simulink model "ModelR3"  (R2020a)
settings: Solver=FixedStepAuto  StartTime=0.0  StopTime=Tf  FixedStep=0.1  RelTol=1e-3
undefined symbols (not defined in the file): amax_ego, amin_ego, d_target, t_gap, Tf, Ts, v0_ego, v0_lead, x0_ego, x0_lead
libraries: simulink x6, rllib x1
settings Model: Creator=The MathWorks, Inc.  LastModifiedBy=kn944
settings DataIOCC: ReturnWorkspaceOutputs=off
settings DebuggingCC: ArithmeticOperatorsInVariantConditions=warning
settings SFSimCC: SimUseLocalCustomCode=off
settings RTWCC: RTWUseLocalCustomCode=off
settings CodeAppCC: StateflowObjectComments=on

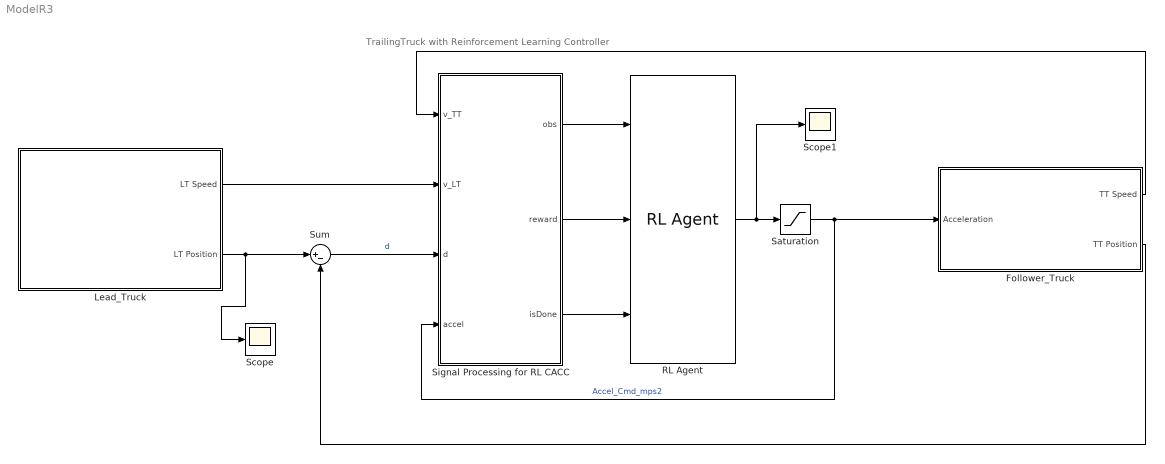
== system ModelR3 ==
  note: TrailingTruck with Reinforcement Learning Controller
  Follower_Truck : Subsystem
  Lead_Truck : Subsystem
  RL Agent : rllib/RL Agent  Agent=agent  ProvideReward=on  ProvideIsDone=on  ProvideCumRwd=off  TreatAsDirectFeedthrough=on  CollectLoggedSignals=on  CollectModelStates=on
  Saturation : Saturate  UpperLimit=amax_ego  LowerLimit=amin_ego
  Scope : Scope
  Scope1 : Scope
  Signal Processing for RL CACC : Subsystem
  Sum : Sum  Inputs=|+-
  wires:
  Signal Processing for RL CACC/2(reward) -> RL Agent/2
  Signal Processing for RL CACC/3(isDone) -> RL Agent/3
  Signal Processing for RL CACC/1(obs) -> RL Agent/1
  Sum/1 -> Signal Processing for RL CACC/3(d)  "d"
  Saturation/1 -> Signal Processing for RL CACC/4(accel), Follower_Truck/1(Acceleration)  "Accel_Cmd_mps2"
  Lead_Truck/1(LT Speed) -> Signal Processing for RL CACC/2(v_LT)
  Lead_Truck/2(LT Position) -> Scope/1, Sum/1
  Follower_Truck/1(TT Speed) -> Signal Processing for RL CACC/1(v_TT)
  Follower_Truck/2(TT Position) -> Sum/2
  RL Agent/1 -> Scope1/1, Saturation/1

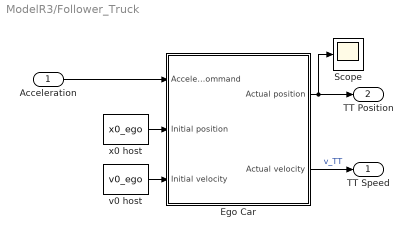
== system ModelR3/Follower_Truck ==
  Acceleration : Inport
  Ego Car : Subsystem
  Scope : Scope
  v0 host : Constant  Value=v0_ego  SampleTime=Ts
  x0 host : Constant  Value=x0_ego  SampleTime=Ts
  TT Speed : Outport
  TT Position : Outport  Port=2
  wires:
  Ego Car/1(Actual position) -> TT Position/1, Scope/1
  x0 host/1 -> Ego Car/2(Initial position)
  v0 host/1 -> Ego Car/3(Initial velocity)
  Ego Car/2(Actual velocity) -> TT Speed/1  "v_TT"
  Acceleration/1 -> Ego Car/1(Acceleration Command)

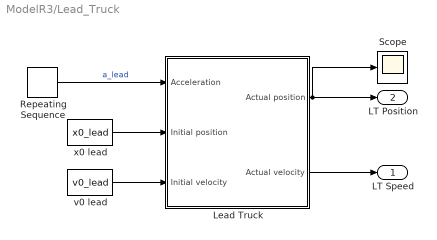
== system ModelR3/Lead_Truck ==
  Lead Truck : Subsystem
  Repeating Sequence : simulink/Sources/Repeating Sequence  rep_seq_t=[0 5 5.1 8 8.1 15 15.1 17 17.1 25]  rep_seq_y=[0 0 0.8 0.8 0 0 -2 -2 0 0]
  Scope : Scope
  v0 lead : Constant  Value=v0_lead  SampleTime=Ts
  x0 lead : Constant  Value=x0_lead  SampleTime=Ts
  LT Speed : Outport
  LT Position : Outport  Port=2
  wires:
  Repeating Sequence/1 -> Lead Truck/1(Acceleration)  "a_lead"
  x0 lead/1 -> Lead Truck/2(Initial position)
  v0 lead/1 -> Lead Truck/3(Initial velocity)
  Lead Truck/2(Actual velocity) -> LT Speed/1
  Lead Truck/1(Actual position) -> Scope/1, LT Position/1

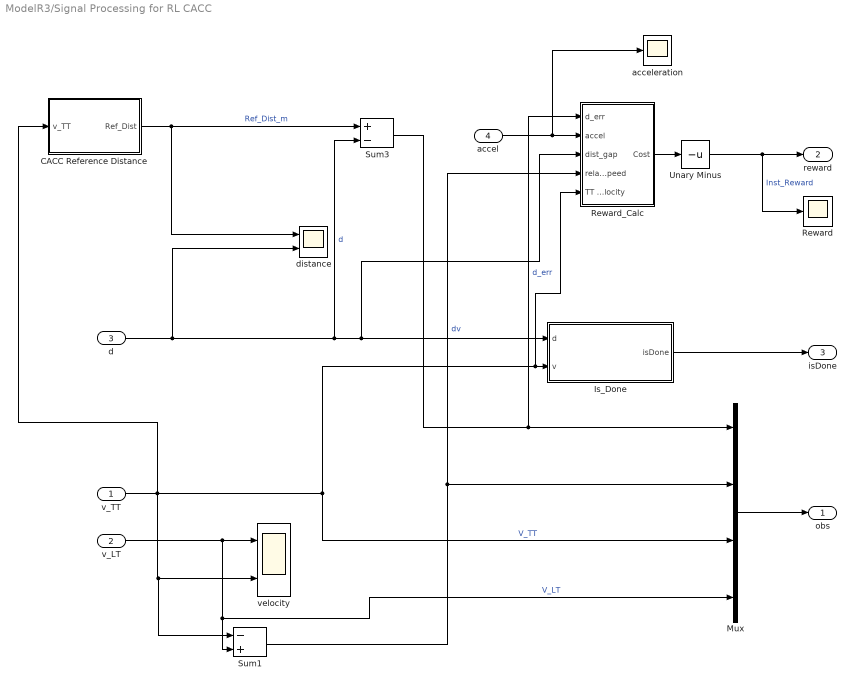
== system ModelR3/Signal Processing for RL CACC ==
  v_TT : Inport
  v_LT : Inport  Port=2
  d : Inport  Port=3
  accel : Inport  Port=4
  CACC Reference Distance : Subsystem
  Is_Done : Subsystem
  Mux : Mux
  Reward : Scope
  Reward_Calc : Subsystem
  Sum1 : Sum  Inputs=-+
  Sum3 : Sum  Inputs=+-
  Unary Minus : UnaryMinus
  acceleration : Scope
  distance : Scope  NumInputPorts=2
  velocity : Scope  NumInputPorts=2
  obs : Outport  VectorParamsAs1DForOutWhenUnconnected=off
  reward : Outport  Port=2  VectorParamsAs1DForOutWhenUnconnected=off
  isDone : Outport  Port=3  VectorParamsAs1DForOutWhenUnconnected=off
  wires:
  Mux/1 -> obs/1
  v_TT/1 -> Sum1/1, velocity/2, Mux/3, Reward_Calc/5(TT velocity), Is_Done/2(v), CACC Reference Distance/1(v_TT)  "V_TT"
  d/1 -> Sum3/2, Reward_Calc/3(dist_gap), Is_Done/1(d), distance/2  "d"
  Reward_Calc/1(Cost) -> Unary Minus/1
  Unary Minus/1 -> Reward/1, reward/1  "Inst_Reward"
  Sum3/1 -> Reward_Calc/1(d_err), Mux/1  "d_err"
  accel/1 -> acceleration/1, Reward_Calc/2(accel)
  Is_Done/1(isDone) -> isDone/1
  CACC Reference Distance/1(Ref_Dist) -> Sum3/1, distance/1  "Ref_Dist_m"
  v_LT/1 -> Mux/4, Sum1/2, velocity/1  "V_LT"
  Sum1/1 -> Reward_Calc/4(relative_Speed), Mux/2  "dv"

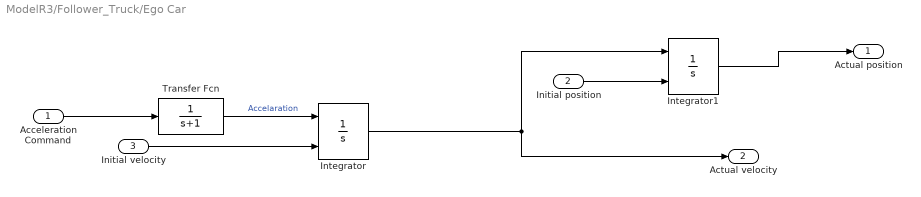
== system ModelR3/Follower_Truck/Ego Car ==
  Acceleration Command : Inport
  Initial position : Inport  Port=2
  Initial velocity : Inport  Port=3
  Integrator : Integrator  InitialConditionSource=external  UpperSaturationLimit=42  LowerSaturationLimit=0
  Integrator1 : Integrator  InitialConditionSource=external  UpperSaturationLimit=500  LowerSaturationLimit=0
  Transfer Fcn : TransferFcn  Denominator=[1 1]
  Actual position : Outport  VectorParamsAs1DForOutWhenUnconnected=off
  Actual velocity : Outport  Port=2  VectorParamsAs1DForOutWhenUnconnected=off
  wires:
  Integrator1/1 -> Actual position/1
  Initial position/1 -> Integrator1/2
  Integrator/1 -> Integrator1/1, Actual velocity/1
  Initial velocity/1 -> Integrator/2
  Transfer Fcn/1 -> Integrator/1  "Accelaration"
  Acceleration Command/1 -> Transfer Fcn/1

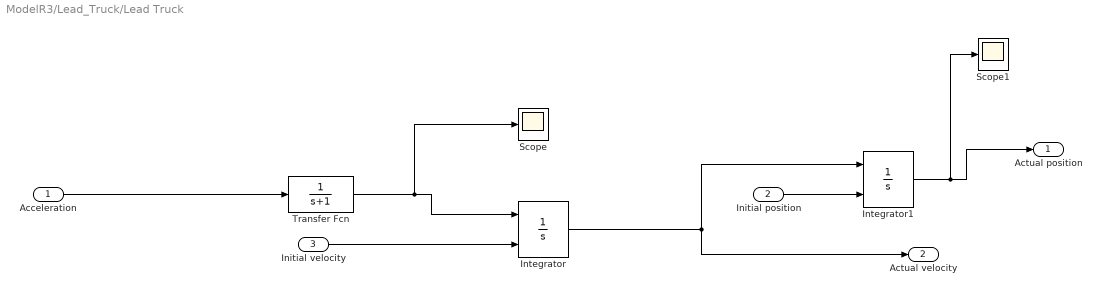
== system ModelR3/Lead_Truck/Lead Truck ==
  Acceleration : Inport
  Initial position : Inport  Port=2
  Initial velocity : Inport  Port=3
  Integrator : Integrator  InitialConditionSource=external  UpperSaturationLimit=40  LowerSaturationLimit=0
  Integrator1 : Integrator  InitialConditionSource=external  UpperSaturationLimit=500  LowerSaturationLimit=0
  Scope : Scope
  Scope1 : Scope
  Transfer Fcn : TransferFcn  Denominator=[1 1]
  Actual position : Outport  VectorParamsAs1DForOutWhenUnconnected=off
  Actual velocity : Outport  Port=2  VectorParamsAs1DForOutWhenUnconnected=off
  wires:
  Integrator1/1 -> Scope1/1, Actual position/1
  Integrator/1 -> Integrator1/1, Actual velocity/1
  Initial velocity/1 -> Integrator/2
  Transfer Fcn/1 -> Scope/1, Integrator/1
  Acceleration/1 -> Transfer Fcn/1
  Initial position/1 -> Integrator1/2

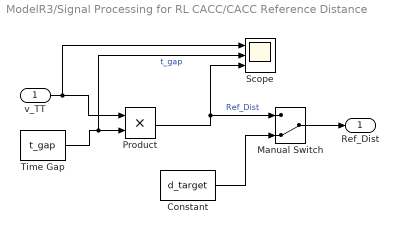
== system ModelR3/Signal Processing for RL CACC/CACC Reference Distance ==
  v_TT : Inport
  Constant : Constant  Value=d_target
  Manual Switch : ManualSwitch  CurrentSetting=0
  Product : Product
  Scope : Scope  NumInputPorts=3
  Time Gap : Constant  Value=t_gap  SampleTime=Ts
  Ref_Dist : Outport  VectorParamsAs1DForOutWhenUnconnected=off
  wires:
  Time Gap/1 -> Scope/2, Product/2  "t_gap"
  Product/1 -> Manual Switch/1, Scope/3  "Ref_Dist"
  v_TT/1 -> Scope/1, Product/1
  Manual Switch/1 -> Ref_Dist/1
  Constant/1 -> Manual Switch/2

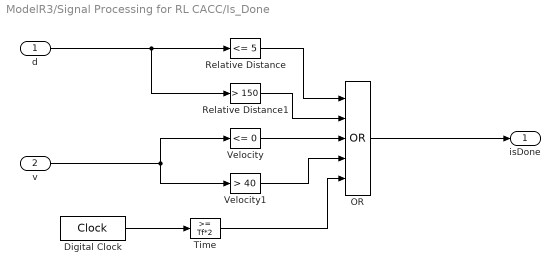
== system ModelR3/Signal Processing for RL CACC/Is_Done ==
  d : Inport
  v : Inport  Port=2
  Digital Clock : DigitalClock
  OR : Logic  Operator=OR  Inputs=5  AllPortsSameDT=off  OutDataTypeStr=boolean
  Relative Distance : simulink/Logic and Bit Operations/Compare To Constant  relop=<=  const=5  OutDataTypeStr=boolean
  Relative Distance1 : simulink/Logic and Bit Operations/Compare To Constant  relop=>  const=150  OutDataTypeStr=boolean
  Time : simulink/Logic and Bit Operations/Compare To Constant  relop=>=  const=Tf*2  OutDataTypeStr=boolean
  Velocity : simulink/Logic and Bit Operations/Compare To Constant  relop=<=  const=0  OutDataTypeStr=boolean
  Velocity1 : simulink/Logic and Bit Operations/Compare To Constant  relop=>  const=40  OutDataTypeStr=boolean
  isDone : Outport  VectorParamsAs1DForOutWhenUnconnected=off
  wires:
  d/1 -> Relative Distance1/1, Relative Distance/1
  v/1 -> Velocity1/1, Velocity/1
  OR/1 -> isDone/1
  Relative Distance/1 -> OR/1
  Relative Distance1/1 -> OR/2
  Velocity/1 -> OR/3
  Velocity1/1 -> OR/4
  Digital Clock/1 -> Time/1
  Time/1 -> OR/5

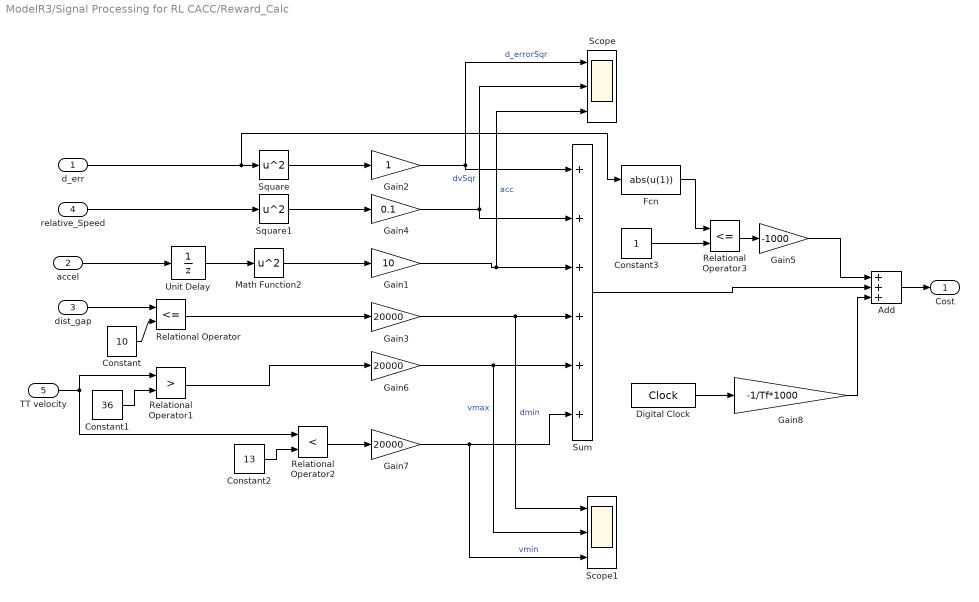
== system ModelR3/Signal Processing for RL CACC/Reward_Calc ==
  d_err : Inport
  accel : Inport  Port=2
  dist_gap : Inport  Port=3
  relative_Speed : Inport  Port=4
  TT velocity : Inport  Port=5
  Add : Sum  Inputs=+++
  Constant : Constant  Value=10
  Constant1 : Constant  Value=36
  Constant2 : Constant  Value=13
  Constant3 : Constant
  Digital Clock : DigitalClock
  Fcn : Fcn  Expr=abs(u(1))
  Gain1 : Gain  Gain=10
  Gain2 : Gain
  Gain3 : Gain  Gain=20000
  Gain4 : Gain  Gain=0.1
  Gain5 : Gain  Gain=-1000
  Gain6 : Gain  Gain=20000
  Gain7 : Gain  Gain=20000
  Gain8 : Gain  Gain=-1/Tf*1000
  Math Function2 : Math  Operator=square  SignedPower=on  SaturateOnIntegerOverflow=on
  Relational Operator : RelationalOperator  Operator=<=  OutDataTypeStr=boolean  RndMeth=Simplest
  Relational Operator1 : RelationalOperator  Operator=>  OutDataTypeStr=boolean  RndMeth=Simplest
  Relational Operator2 : RelationalOperator  Operator=<  OutDataTypeStr=boolean  RndMeth=Simplest
  Relational Operator3 : RelationalOperator  Operator=<=  OutDataTypeStr=boolean  RndMeth=Simplest
  Scope : Scope  NumInputPorts=3
  Scope1 : Scope  NumInputPorts=3
  Square : Math  Operator=square  SignedPower=on  SaturateOnIntegerOverflow=on
  Square1 : Math  Operator=square  SignedPower=on  SaturateOnIntegerOverflow=on
  Sum : Sum  Inputs=++++++
  Unit Delay : UnitDelay  SampleTime=-1  HasFrameUpgradeWarning=on
  Cost : Outport  VectorParamsAs1DForOutWhenUnconnected=off
  wires:
  d_err/1 -> Fcn/1, Square/1
  Math Function2/1 -> Gain1/1
  Square/1 -> Gain2/1
  accel/1 -> Unit Delay/1
  dist_gap/1 -> Relational Operator/1
  Constant/1 -> Relational Operator/2
  Relational Operator/1 -> Gain3/1
  relative_Speed/1 -> Square1/1
  Square1/1 -> Gain4/1
  Gain2/1 -> Scope/1, Sum/1  "d_errorSqr"
  Gain4/1 -> Scope/2, Sum/2  "dvSqr"
  Unit Delay/1 -> Math Function2/1
  Relational Operator1/1 -> Gain6/1
  Constant1/1 -> Relational Operator1/2
  Relational Operator2/1 -> Gain7/1
  Constant2/1 -> Relational Operator2/2
  TT velocity/1 -> Relational Operator2/1, Relational Operator1/1
  Gain7/1 -> Scope1/3, Sum/6  "vmin"
  Gain1/1 -> Scope/3, Sum/3  "acc"
  Gain3/1 -> Scope1/1, Sum/4  "dmin"
  Gain6/1 -> Scope1/2, Sum/5  "vmax"
  Sum/1 -> Add/2
  Add/1 -> Cost/1
  Constant3/1 -> Relational Operator3/2
  Fcn/1 -> Relational Operator3/1
  Relational Operator3/1 -> Gain5/1
  Gain5/1 -> Add/1
  Digital Clock/1 -> Gain8/1
  Gain8/1 -> Add/3
